simulink model "OADP_example"  (R2021a)
settings: Solver=VariableStepAuto  StartTime=0.0  StopTime=10  RelTol=1e-3
settings Model: Creator=ADMIN  LastModifiedBy=ADMIN

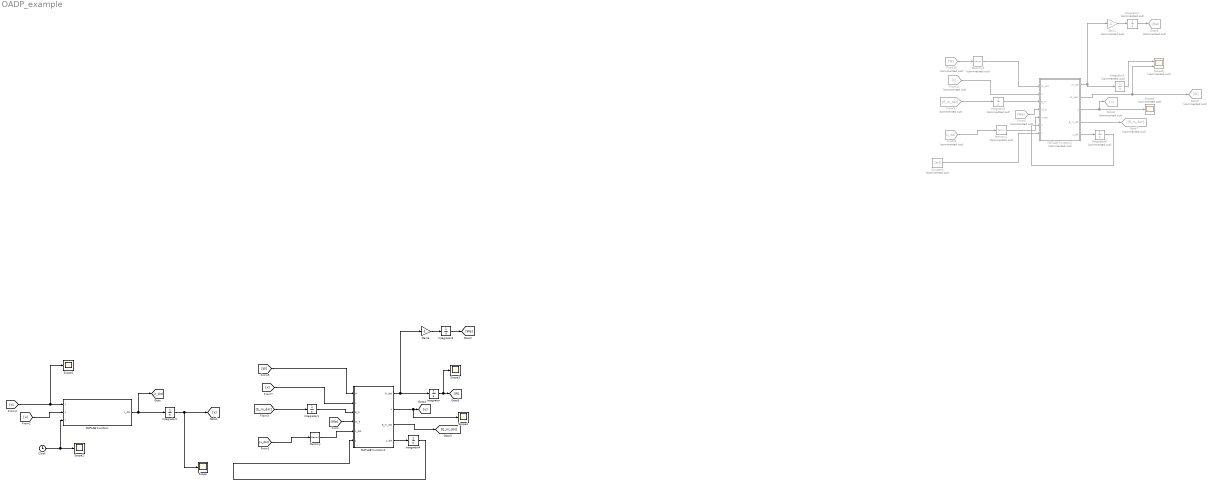
== system OADP_example ==
  Clock : Clock
  Constant : Constant  Commented=on  Value=1e-6
  From10 : From  Commented=on  GotoTag=W
  From11 : From  Commented=on  GotoTag=x
  From6 : From  Commented=on  GotoTag=We
  From8 : From  Commented=on  GotoTag=x_dot
  From9 : From  Commented=on  GotoTag=E_m_dot
  Gain1 : Gain  Commented=on  Gain=-1
  Gain6 : Gain  Gain=-1
  Goto6 : Goto  Commented=on  GotoTag=We
  Goto7 : Goto  Commented=on  GotoTag=E_m_dot
  Goto8 : Goto  Commented=on  GotoTag=u
  Goto9 : Goto  Commented=on  GotoTag=W
  Integrator : Integrator  InitialCondition=[0.4, 0.5, 1.6, 0.2, 1.8, 0.3, 1.2, 1, 0.7, 1.5]'
  Integrator1 : Integrator
  Integrator2 : Integrator  InitialCondition=[1; 0.5;-1;-0.5]
  Integrator3 : Integrator  InitialCondition=[0;0;0;0;0;0;0;0;0;0]
  Integrator4 : Integrator  InitialCondition=[0;0;0;0]
  Integrator5 : Integrator  Commented=on  InitialCondition=[0.4, 0.5, 1.6, 0.2, 1.8, 0.3, 1.2, 1, 0.7, 1.5]'
  Integrator6 : Integrator  Commented=on
  Integrator7 : Integrator  Commented=on  InitialCondition=[0;0;0;0;0;0;0;0;0;0]
  Integrator8 : Integrator  Commented=on  InitialCondition=[0;0;0;0]
  MATLAB Function : MATLAB Function  TreatAsAtomicUnit=on
  MATLAB Function1 : MATLAB Function  TreatAsAtomicUnit=on
  MATLAB Function2 : MATLAB Function  Commented=on  TreatAsAtomicUnit=on
  Memory : Memory  InitialCondition=[0;0;0;0]
  Memory1 : Memory  Commented=on  InitialCondition=[0;0;0;0]
  Memory2 : Memory  Commented=on  InitialCondition=[0.4, 0.5, 1.6, 0.2, 1.8, 0.3, 1.2, 1, 0.7, 1.5]'
  Scope{,1..4} (5 alike) : Scope
  Scope5 : Scope  Commented=on  NumInputPorts=2
  Scope6 : Scope  Commented=on
  wires:
  [W] -> MATLAB Function1/1(W)
  [E_m_dot] -> Integrator1/1
  MATLAB Function1/3(E_m_dot) -> [E_m_dot]
  Gain6/1 -> Integrator3/1
  Integrator/1 -> Scope3/1, [W]
  MATLAB Function1/2(u) -> Scope4/1, [u]
  Integrator2/1 -> Scope/1, [x]
  [u] -> MATLAB Function/2(u)
  [x] -> MATLAB Function1/2(x)
  MATLAB Function/1(x_dot) -> Integrator2/1, [x_dot]
  MATLAB Function1/1(W_dot) -> Gain6/1, Integrator/1
  Clock/1 -> MATLAB Function/3(t), Scope2/1
  MATLAB Function1/4(z_dot) -> Integrator4/1
  Integrator4/1 -> MATLAB Function1/6(z)
  Integrator1/1 -> MATLAB Function1/3(E_m)
  Integrator3/1 -> [We]
  [We] -> MATLAB Function1/4(W_e)
  [x] -> Scope1/1, MATLAB Function/1(x)
  Memory/1 -> MATLAB Function1/5(x_dot)
  [x_dot] -> Memory/1
  Integrator8/1 -> MATLAB Function2/6(z)
  MATLAB Function2/5(z_dot) -> Integrator8/1
  Gain1/1 -> Integrator7/1
  Integrator6/1 -> MATLAB Function2/3(E_m)
  Integrator7/1 -> Goto6/1
  From6/1 -> MATLAB Function2/4(W_e)
  Memory1/1 -> MATLAB Function2/5(x_dot)
  MATLAB Function2/4(E_m_dot) -> Goto7/1
  MATLAB Function2/1(W_dot) -> Integrator5/1, Gain1/1
  From9/1 -> Integrator6/1
  MATLAB Function2/3(u) -> Goto8/1, Scope6/1
  From8/1 -> Memory1/1
  Integrator5/1 -> Scope5/1
  From11/1 -> MATLAB Function2/2(x)
  MATLAB Function2/2(W_new) -> Scope5/2, Goto9/1
  From10/1 -> Memory2/1
  Memory2/1 -> MATLAB Function2/1(W_old)
  Constant/1 -> MATLAB Function2/7(t)

== matlab function OADP_example/MATLAB Function1 ==
  data: W input; W_dot output; x input; E_m input; W_e input; x_dot input; u output; E_m_dot output; z input; z_dot output
function [W_dot, u, E_m_dot, z_dot] = fcn(W, x, E_m, W_e, x_dot,z)
%% parameter
 f =  [x(2)-x(1); 
      -0.5*(x(1)+x(2)) + 0.5*x(2)*(cos(2*x(1))+2)^2; 
      x(4)-x(3); 
      -x(3)-0.5*x(4)+0.5*(x(3)^2)*x(4)];
 g = [0 0; 
      cos(2*x(1))+2 0; 
      0 0; 
      0 x(3)+2*exp(-x(4))];
%% set up
 K = 10*eye(4);
 R = eye(2);
 Q = eye(4);
 I_c = 0.1;
 I_e = 0.1;
 nuy = 1;
 Grad_Sigma = [2*x(1) 0 0 0; 
               x(2) x(1) 0 0; 
               x(3) 0 x(1) 0; 
               x(4) 0 0 x(1); 
               0 2*x(2) 0 0; 
               0 x(3) x(2) 0; 
               0 x(4) 0 x(2); 
               0 0 2*x(3) 0; 
               0 0 x(4) x(3); 
               0 0 0 2*x(4)];
 theta = Grad_Sigma*x_dot;
 Grad_V = Grad_Sigma'*W;
 
%% update u
u = -(1/2)*R'*g'*Grad_Sigma'*W;

%% observer
d_mu = K*(x-z);
z_dot = f + g*u + d_mu + K*x;

%% update W

E_c = norm(d_mu)*norm(Grad_V') + x'*Q*x + u'*R*u+ W'*theta;
E_m_dot = -I_e*W'*theta;
W_dot = -I_c*(E_c - E_m - nuy*sign(W_e'*theta))*theta;
%{
E_c = x'*Q*x + u'*R*u+ W'*theta;
E_m_dot = -I_e*W'*theta;
W_dot = -I_c*(E_c - E_m - nuy*sign(W_e'*theta))*theta;
%}
end

== matlab function OADP_example/MATLAB Function ==
  data: x input; x_dot output; u input; t input
function x_dot = fcn(x, u, t)
 f =  [x(2)-x(1); 
      -0.5*(x(1)+x(2)) + 0.5*x(2)*(cos(2*x(1))+2)^2; 
      x(4)-x(3); 
      -x(3)-0.5*x(4)+0.5*(x(3)^2)*x(4)];
 g = [0 0; 
      cos(2*x(1))+2 0; 
      0 0; 
      0 x(3)+2*exp(-x(4))];
 z = [0.6*x(1)*cos(x(2)*x(3)); 
      0.05*x(2)*x(3)*cos(x(4)^2); 
      0.15*x(4)*cos(pi*t)*cos(x(3)+x(4)); 
      0.4*x(4)*sin(3*pi*t)*exp(-2*x(2))];
 d = 0.2*f + 0.15*g*u + z;
 x_dot = f + g*u +d;
end

== matlab function OADP_example/MATLAB Function2 ==
  data: W_dot output; W_new output; W_old input; x input; E_m input; W_e input; x_dot input; z input; u output; E_m_dot output; t input; z_dot output
function [W_dot,W_new, u, E_m_dot, z_dot] = fcn(W_old, x, E_m, W_e, x_dot,z, t)
%% parameter
 f =  [x(2)-x(1); 
      -0.5*(x(1)+x(2)) + 0.5*x(2)*(cos(2*x(1))+2)^2; 
      x(4)-x(3); 
      -x(3)-0.5*x(4)+0.5*(x(3)^2)*x(4)];
 g = [0 0; 
      cos(2*x(1))+2 0; 
      0 0; 
      0 x(3)+2*exp(-x(4))];
%% set up
 K = 10*eye(4);
 R = eye(2);
 Q = eye(4);
 I_c = 0.1;
 I_e = 0.1;
 nuy = 1;
 Grad_Sigma = [2*x(1) 0 0 0; 
               x(2) x(1) 0 0; 
               x(3) 0 x(1) 0; 
               x(4) 0 0 x(1); 
               0 2*x(2) 0 0; 
               0 x(3) x(2) 0; 
               0 x(4) 0 x(2); 
               0 0 2*x(3) 0; 
               0 0 x(4) x(3); 
               0 0 0 2*x(4)];
 theta = Grad_Sigma*x_dot;
 Grad_V = Grad_Sigma'*W_old;
 
%% update u
u = -(1/2)*R'*g'*Grad_Sigma'*W_old;

%% observer
d_mu = K*(x-z);
z_dot = f + g*u + d_mu + K*x;

%% update W

E_c = norm(d_mu)*norm(Grad_V') + x'*Q*x + u'*R*u+ W_old'*theta;
E_m_dot = -I_e*W_old'*theta;
W_dot = -I_c*(E_c - E_m - nuy*sign(W_e'*theta))*theta;

W_new = W_old + W_dot*t;
%{
E_c = x'*Q*x + u'*R*u+ W'*theta;
E_m_dot = -I_e*W'*theta;
W_dot = -I_c*(E_c - E_m - nuy*sign(W_e'*theta))*theta;
%}
end
